simulink model "City_Env_2Car_CS2020"  (Simulink 8.8)
settings: Solver=ode45  StartTime=0  StopTime=20  RelTol=1e-3  EnableMultiTasking=on
libraries: Solver_SF x2
settings Model: Creator=dhall  LastModifiedBy=mkhan  ExtModeTrigMode=oneshot  ExtModeArmWhenConnect=off
settings DataIOCC: LimitDataPoints=off  SignalLoggingName=sigsOut
settings OptimizationCC: BooleanDataType=off  LocalBlockOutputs=off  InitFltsAndDblsToZero=on
settings DebuggingCC: SaveWithParameterizedLinksMsg=none  SignalResolutionControl=TryResolveAllWithWarning  MultiTaskDSMMsg=warning  MultiTaskCondExecSysMsg=none  SFExecutionAtInitializationDiag=warning
settings HardwareCC: TargetUnknown=on
settings GRTTargetCC: TargetFcnLib=ansi_tfl_tmw.mat  CompOptLevelCompliant=off
settings ConfigComp: CovSFcnEnable=off

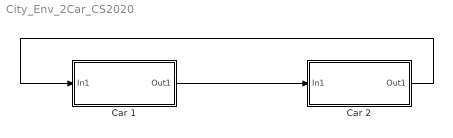
== system City_Env_2Car_CS2020 ==
  Car 1 : Subsystem
  Car 2 : Subsystem
  wires:
  Car 1/1(Out1) -> Car 2/1(In1)
  Car 2/1(Out1) -> Car 1/1(In1)

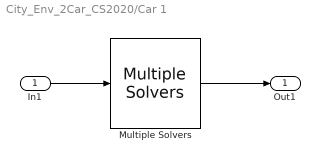
== system City_Env_2Car_CS2020/Car 1 ==
  In1 : Inport
  Multiple Solvers : Solver_SF/Multiple Solvers  Priority=1  iVehicle=1  SIMFILE=D:\mech_sim\trunk\Image\CarSim\Core\CarSim_Data\Extensions\Simulink\Multi_Vehicle\simfile1.sim  Run_RTs=off  vs_state_ind=Run  StopMode_ind=Vehicle Model  vs_scx=on
  Out1 : Outport
  wires:
  In1/1 -> Multiple Solvers/1
  Multiple Solvers/1 -> Out1/1

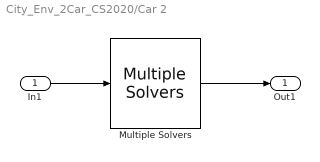
== system City_Env_2Car_CS2020/Car 2 ==
  In1 : Inport
  Multiple Solvers : Solver_SF/Multiple Solvers  Priority=1  iVehicle=2  SIMFILE=D:\mech_sim\trunk\Image\CarSim\Core\CarSim_Data\Extensions\Simulink\Multi_Vehicle\simfile2.sim  Run_RTs=off  vs_state_ind=Run  StopMode_ind=Vehicle Model  vs_scx=on
  Out1 : Outport
  wires:
  In1/1 -> Multiple Solvers/1
  Multiple Solvers/1 -> Out1/1
